simulink model "double_source_V3"  (R2023a)
settings: Solver=ode23tb  StartTime=0.0  StopTime=1  MaxStep=1e-6  RelTol=1e-3
libraries: spsSeriesRLCBranchLib x11, spsGroundLib x8, spsMosfetLib x8, spsVoltageMeasurementLib x4, spsACVoltageSourceLib x3, spsCurrentMeasurementLib x2, simulink x2, sps_lib x1
settings Model: Creator=25417  LastModifiedBy=25417

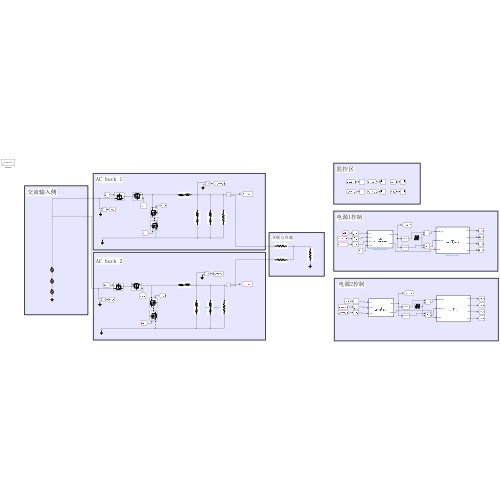
[thumbnail: Simulink's stored preview of the top-level diagram]
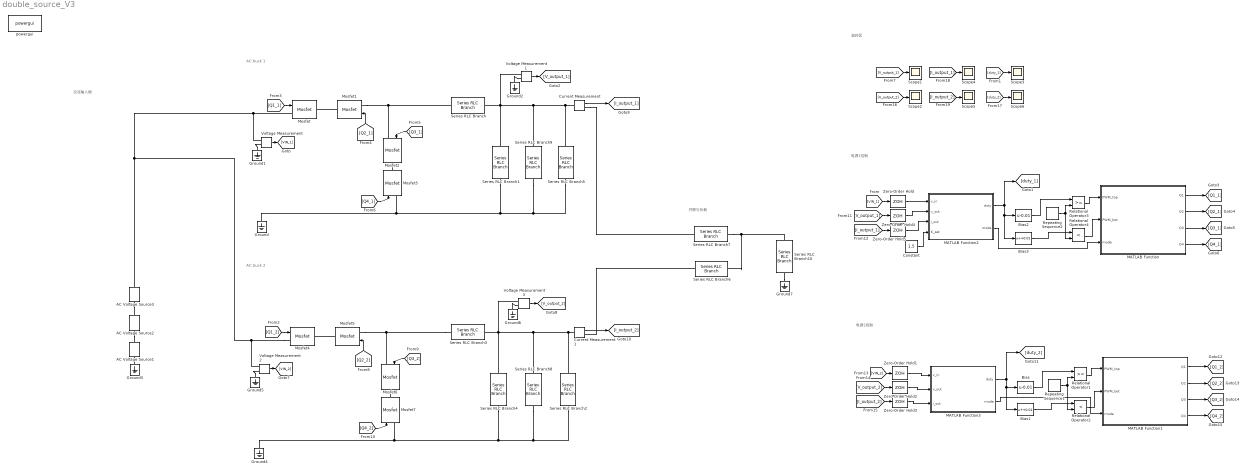
== system double_source_V3 ==
  note: 监控区
  note: 电源1控制
  note: 并联与负载
  note: AC buck 1
  note: 交流输入侧
  note: AC buck 2
  note: 电源2控制
  AC Voltage Source1 : spsACVoltageSourceLib/AC Voltage Source  Amplitude=70  Phase=0  Frequency=50  SampleTime=0  Measurements=None  BusType=swing  Pref=10e3  Qref=0  Qmin=-inf  Qmax=+inf
  AC Voltage Source2 : spsACVoltageSourceLib/AC Voltage Source  Amplitude=2.1  Phase=180  Frequency=150  SampleTime=0  Measurements=None  BusType=swing  Pref=10e3  Qref=0  Qmin=-inf  Qmax=+inf
  AC Voltage Source3 : spsACVoltageSourceLib/AC Voltage Source  Amplitude=1.4  Phase=180  Frequency=250  SampleTime=0  Measurements=None  BusType=swing  Pref=10e3  Qref=0  Qmin=-inf  Qmax=+inf
  Bias : Bias  Bias=-0.01  SaturateOnIntegerOverflow=off
  Bias1 : Bias  Bias=+0.01  SaturateOnIntegerOverflow=off
  Bias2 : Bias  Bias=-0.01  SaturateOnIntegerOverflow=off
  Bias3 : Bias  Bias=+0.01  SaturateOnIntegerOverflow=off
  Constant : Constant  Value=1.5
  Current Measurement : spsCurrentMeasurementLib/Current Measurement  PhasorSimulation=off  OutputType=Complex  PSBequivalent=0
  Current Measurement1 : spsCurrentMeasurementLib/Current Measurement  PhasorSimulation=off  OutputType=Complex  PSBequivalent=0
  Ground{,1..7} (8 alike) : spsGroundLib/Ground  LConnTagsString=a
  MATLAB Function : MATLAB Function  TreatAsAtomicUnit=on  SystemSampleTime=0
  MATLAB Function1 : MATLAB Function  TreatAsAtomicUnit=on  SystemSampleTime=0
  MATLAB Function2 : MATLAB Function  TreatAsAtomicUnit=on  SystemSampleTime=1/20e3
  MATLAB Function3 : MATLAB Function  TreatAsAtomicUnit=on  SystemSampleTime=1/20e3
  Mosfet{,1..7} (8 alike) : spsMosfetLib/Mosfet  Ron=0.1  Lon=0  Rd=0.01  Vfd=0  IC=0  Rs=1e5  Cs=inf  Measurements=off
  Relational Operator1 : RelationalOperator  OutDataTypeStr=boolean  RndMeth=Simplest  InputSameDT=off
  Relational Operator2 : RelationalOperator  Operator=<  OutDataTypeStr=boolean  RndMeth=Simplest  InputSameDT=off
  Relational Operator3 : RelationalOperator  OutDataTypeStr=boolean  RndMeth=Simplest  InputSameDT=off
  Relational Operator4 : RelationalOperator  Operator=<  OutDataTypeStr=boolean  RndMeth=Simplest  InputSameDT=off
  Repeating Sequence1 : simulink/Sources/Repeating Sequence  rep_seq_t=[0, 1/20000]  rep_seq_y=[0 1]
  Repeating Sequence2 : simulink/Sources/Repeating Sequence  rep_seq_t=[0, 1/20000]  rep_seq_y=[0 1]
  Scope{1..6} (6 alike) : Scope
  Series RLC Branch : spsSeriesRLCBranchLib/Series RLC Branch  LConnTagsString=__new0  RConnTagsString=__new0  BranchType=RL  Resistance=0.04  Inductance=450e-6  SetiL0=off  InitialCurrent=0  Capacitance=1e-6  Setx0=off  InitialVoltage=0  Measurements=None
  Series RLC Branch1 : spsSeriesRLCBranchLib/Series RLC Branch  LConnTagsString=__new0  RConnTagsString=__new0  BranchType=RC  Resistance=0.01  Inductance=1e-3  SetiL0=off  InitialCurrent=0  Capacitance=10.34e-6  Setx0=off  InitialVoltage=0  Measurements=None
  Series RLC Branch10 : spsSeriesRLCBranchLib/Series RLC Branch  LConnTagsString=__new0  RConnTagsString=__new0  BranchType=R  Resistance=10  Inductance=1e-3  SetiL0=off  InitialCurrent=0  Capacitance=10e-6  Setx0=off  InitialVoltage=0  Measurements=None
  Series RLC Branch2 : spsSeriesRLCBranchLib/Series RLC Branch  LConnTagsString=__new0  RConnTagsString=__new0  BranchType=R  Resistance=1.93e3  Inductance=1e-3  SetiL0=off  InitialCurrent=0  Capacitance=2e4  Setx0=off  InitialVoltage=0  Measurements=None
  Series RLC Branch3 : spsSeriesRLCBranchLib/Series RLC Branch  LConnTagsString=__new0  RConnTagsString=__new0  BranchType=RL  Resistance=0.07  Inductance=490e-6  SetiL0=off  InitialCurrent=0  Capacitance=1e-6  Setx0=off  InitialVoltage=0  Measurements=None
  Series RLC Branch4 : spsSeriesRLCBranchLib/Series RLC Branch  LConnTagsString=__new0  RConnTagsString=__new0  BranchType=RC  Resistance=0.01  Inductance=1e-3  SetiL0=off  InitialCurrent=0  Capacitance=9.54e-6  Setx0=off  InitialVoltage=0  Measurements=None
  Series RLC Branch5 : spsSeriesRLCBranchLib/Series RLC Branch  LConnTagsString=__new0  RConnTagsString=__new0  BranchType=R  Resistance=2.1e3  Inductance=1e-3  SetiL0=off  InitialCurrent=0  Capacitance=2e4  Setx0=off  InitialVoltage=0  Measurements=None
  Series RLC Branch6 : spsSeriesRLCBranchLib/Series RLC Branch  LConnTagsString=__new0  RConnTagsString=__new0  BranchType=R  Resistance=0.01  Inductance=1e-3  SetiL0=off  InitialCurrent=0  Capacitance=10e-6  Setx0=off  InitialVoltage=0  Measurements=None
  Series RLC Branch7 : spsSeriesRLCBranchLib/Series RLC Branch  LConnTagsString=__new0  RConnTagsString=__new0  BranchType=R  Resistance=0.01  Inductance=1e-3  SetiL0=off  InitialCurrent=0  Capacitance=10e-6  Setx0=off  InitialVoltage=0  Measurements=None
  Series RLC Branch8 : spsSeriesRLCBranchLib/Series RLC Branch  LConnTagsString=__new0  RConnTagsString=__new0  BranchType=RC  Resistance=0.01  Inductance=1e-3  SetiL0=off  InitialCurrent=0  Capacitance=4.5e-6  Setx0=off  InitialVoltage=0  Measurements=None
  Series RLC Branch9 : spsSeriesRLCBranchLib/Series RLC Branch  LConnTagsString=__new0  RConnTagsString=__new0  BranchType=RC  Resistance=0.01  Inductance=1e-3  SetiL0=off  InitialCurrent=0  Capacitance=4.81e-6  Setx0=off  InitialVoltage=0  Measurements=None
  Voltage Measurement{,1..3} (4 alike) : spsVoltageMeasurementLib/Voltage Measurement  PhasorSimulation=off  OutputType=Complex  PSBequivalent=0
  Zero-Order Hold{,1..5} (6 alike) : ZeroOrderHold  SampleTime=1/2e4
  powergui : sps_lib/powergui  Priority=1  SimulationMode=Continuous  SampleTime=5e-7  frequency=60  Iterations=50  frequencyindice=50  Pbase=100e6  ErrMax=1e-4  UnitsV=kV  UnitsW=MW  buscounter=0  FunctionMessages=off  echomessages=off  EnableUseOfTLC=off  CurrentSourceSwitches=off  DisableSnubberDevices=off  DisableRonSwitches=off  DisableVfSwitches=off  DisplayEquations=off  AutomaticDiscreteSolvers=off  SolverType=Tustin/Backward Euler (TBE)  Interpol=off  ExternalGateDelay=off  methode=off  Ts=100  x0status=blocks  SPID=on  SwTol=0  HookPort=off  NonlinearTolerance=1e-4  nMaxIteration=100  ContinueOnMaxIteration=off  RestoreLinks=warning  ResistiveCurrentMeasurement=off  Frange=[0:2:500]  Ylog=off  Xlog=on  ShowGrid=off  save=off  variable=ZData  structure=0  ZoomFFT=off  StartTime=0.0  cycles=1  DisplayStyle=1  fundamental=60  FreqAxis=off  MaxFrequency=1000  frequencyindicesteady=1  RmsSteady=1  display=off
  wires:
  Voltage Measurement/1 -> [VIN_1]
  [VIN_1] -> Zero-Order Hold/1
  Voltage Measurement1/1 -> [V_output_1]
  [Q1_1] -> Mosfet/1
  [Q2_1] -> Mosfet1/1
  [Q3_1] -> Mosfet2/1
  [Q4_1] -> Mosfet3/1
  [V_output_1] -> Scope1/1
  Zero-Order Hold/1 -> MATLAB Function2/1(v_in)
  [Q4_2] -> Mosfet7/1
  [Q3_2] -> Mosfet6/1
  [Q2_2] -> Mosfet5/1
  [Q1_2] -> Mosfet4/1
  Voltage Measurement3/1 -> [V_output_2]
  Voltage Measurement2/1 -> [VIN_2]
  Current Measurement/1 -> [I_output_1]
  Current Measurement1/1 -> [I_output_2]
  Relational Operator1/1 -> MATLAB Function1/1(PWM_top)
  Zero-Order Hold1/1 -> MATLAB Function3/1(v_in)
  [VIN_2] -> Zero-Order Hold1/1
  MATLAB Function3/1(duty) -> [duty_2], Bias1/1, Bias/1
  [V_output_2] -> Scope2/1
  [V_output_2] -> Zero-Order Hold2/1
  [I_output_2] -> Zero-Order Hold3/1
  Zero-Order Hold3/1 -> MATLAB Function3/3(i_out)
  Zero-Order Hold2/1 -> MATLAB Function3/2(v_out)
  [V_output_1] -> Zero-Order Hold4/1
  [I_output_1] -> Zero-Order Hold5/1
  Zero-Order Hold4/1 -> MATLAB Function2/2(v_out)
  Zero-Order Hold5/1 -> MATLAB Function2/3(i_out)
  [I_output_1] -> Scope4/1
  [I_output_2] -> Scope5/1
  [duty_1] -> Scope3/1
  [duty_2] -> Scope6/1
  Bias/1 -> Relational Operator1/1
  Bias1/1 -> Relational Operator2/1
  Repeating Sequence1/1 -> Relational Operator2/2, Relational Operator1/2
  Relational Operator2/1 -> MATLAB Function1/2(PWM_bot)
  MATLAB Function1/1(Q1) -> [Q1_2]
  MATLAB Function1/2(Q2) -> [Q2_2]
  MATLAB Function1/3(Q3) -> [Q3_2]
  MATLAB Function1/4(Q4) -> [Q4_2]
  Relational Operator4/1 -> MATLAB Function/2(PWM_bot)
  Bias2/1 -> Relational Operator3/1
  Bias3/1 -> Relational Operator4/1
  MATLAB Function2/1(duty) -> Bias3/1, Bias2/1, [duty_1]
  Repeating Sequence2/1 -> Relational Operator4/2, Relational Operator3/2
  Relational Operator3/1 -> MATLAB Function/1(PWM_top)
  MATLAB Function/1(Q1) -> [Q1_1]
  MATLAB Function/2(Q2) -> [Q2_1]
  MATLAB Function/3(Q3) -> [Q3_1]
  MATLAB Function/4(Q4) -> [Q4_1]
  MATLAB Function3/2(mode) -> MATLAB Function1/3(mode)
  MATLAB Function2/2(mode) -> MATLAB Function/3(mode)
  Constant/1 -> MATLAB Function2/4(K_set)
  connections:
  Mosfet1/RConn1 -- Mosfet/RConn1
  Mosfet1/LConn1 -- Mosfet2/LConn1 -- Series RLC Branch/LConn1
  Mosfet3/RConn1 -- Mosfet2/RConn1
  Mosfet3/LConn1 -- Series RLC Branch5/RConn1 -- Series RLC Branch9/RConn1 -- Series RLC Branch1/RConn1 -- Ground/LConn1
  Series RLC Branch1/LConn1 -- Current Measurement/LConn1 -- Series RLC Branch5/LConn1 -- Series RLC Branch9/LConn1 -- Voltage Measurement1/LConn1 -- Series RLC Branch/RConn1
  Voltage Measurement/LConn2 -- Ground1/LConn1
  Ground2/LConn1 -- Voltage Measurement1/LConn2
  Ground3/LConn1 -- AC Voltage Source1/LConn1
  Mosfet4/LConn1 -- Voltage Measurement2/LConn1 -- AC Voltage Source3/RConn1 -- Voltage Measurement/LConn1 -- Mosfet/LConn1
  Mosfet7/LConn1 -- Series RLC Branch2/RConn1 -- Series RLC Branch8/RConn1 -- Series RLC Branch4/RConn1 -- Ground4/LConn1
  Series RLC Branch3/LConn1 -- Mosfet5/LConn1 -- Mosfet6/LConn1
  Series RLC Branch4/LConn1 -- Series RLC Branch2/LConn1 -- Current Measurement1/LConn1 -- Series RLC Branch8/LConn1 -- Voltage Measurement3/LConn1 -- Series RLC Branch3/RConn1
  Voltage Measurement2/LConn2 -- Ground5/LConn1
  Mosfet7/RConn1 -- Mosfet6/RConn1
  Mosfet5/RConn1 -- Mosfet4/RConn1
  Ground6/LConn1 -- Voltage Measurement3/LConn2
  Series RLC Branch7/RConn1 -- Series RLC Branch10/LConn1 -- Series RLC Branch6/RConn1
  Series RLC Branch10/RConn1 -- Ground7/LConn1
  Current Measurement/RConn1 -- Series RLC Branch7/LConn1
  AC Voltage Source2/LConn1 -- AC Voltage Source1/RConn1
  AC Voltage Source3/LConn1 -- AC Voltage Source2/RConn1
  Series RLC Branch6/LConn1 -- Current Measurement1/RConn1

== matlab function double_source_V3/MATLAB Function1 ==
  data: Q1 output; PWM_top input; Q2 output; Q3 output; Q4 output; PWM_bot input; mode input
function [Q1, Q2, Q3, Q4] = Hardware_Router(PWM_top, PWM_bot, mode)
    pwm_t = double(PWM_top);
    pwm_b = double(PWM_bot);
    
    if mode == 1.0
        % ------------------------------------------------------
        % 正半周：打通下桥臂续流
        % ------------------------------------------------------
        Q1 = pwm_t;  
        Q2 = 1.0;    
        Q3 = pwm_b;  
        Q4 = 1.0;    
    elseif mode == -1.0
        % ------------------------------------------------------
        % 负半周：打通上桥臂续流
        % ------------------------------------------------------
        Q1 = 1.0;    
        Q2 = pwm_t;  
        Q3 = 1.0;    
        Q4 = pwm_b;  
    else
        % ------------------------------------------------------
        % 🌟 mode == 0.0：掉电封锁或死区跨越，全局安全关断
        % ------------------------------------------------------
        Q1 = 0.0;
        Q2 = 0.0;
        Q3 = 0.0;
        Q4 = 0.0;
    end
end

== matlab function double_source_V3/MATLAB Function ==
  data: Q1 output; PWM_top input; Q2 output; Q3 output; Q4 output; PWM_bot input; mode input
function [Q1, Q2, Q3, Q4] = Hardware_Router(PWM_top, PWM_bot, mode)
    pwm_t = double(PWM_top);
    pwm_b = double(PWM_bot);
    
    if mode == 1.0
        % ------------------------------------------------------
        % 正半周：打通下桥臂续流
        % ------------------------------------------------------
        Q1 = pwm_t;  
        Q2 = 1.0;    
        Q3 = pwm_b;  
        Q4 = 1.0;    
    elseif mode == -1.0
        % ------------------------------------------------------
        % 负半周：打通上桥臂续流
        % ------------------------------------------------------
        Q1 = 1.0;    
        Q2 = pwm_t;  
        Q3 = 1.0;    
        Q4 = pwm_b;  
    else
        % ------------------------------------------------------
        % 🌟 mode == 0.0：掉电封锁或死区跨越，全局安全关断
        % ------------------------------------------------------
        Q1 = 0.0;
        Q2 = 0.0;
        Q3 = 0.0;
        Q4 = 0.0;
    end
end

== matlab function double_source_V3/MATLAB Function2 ==
  data: v_in input; v_out input; i_out input; duty output; mode output; K_set input
function [duty, mode] = MCU_ISR_Master(v_in, v_out, i_out, K_set)
    % ==========================================================
    % [1] 用户接口与基础配置区
    % ==========================================================
    % 系统的绝对参考基准电压（有效值）
    % 设定值为后续所有调压、下垂计算的物理锚点。
    V_TARGET_RMS = 30.0; 
    
    % ==========================================================
    % [2] 闭环调参区
    % ==========================================================
    % 基础下垂系数：定义无通讯并联系统的基准输出阻抗
    % 主从机必须保持一致，它是电流反比分配定律的数学基石。
    BASE_DROOP    = 0.55;     
    
    % 电压 PI 环参数配置
    % 本架构属于“前馈主导 + PI辅助”的包络线控制。
    % 较低的比例(Kp)和积分(Ki)旨在只消除硬件线路(DCR/ESR)带来的稳态误差，
    % 避免由于强积分导致控制环路对谐波产生过激反应。
    KP_V          = 0.05;    
    KI_V          = 100.0;    
    
    % 硬件高频噪声低通滤波器系数 (用于平滑 ADC 原始采样值)
    ALPHA_LPF     = 0.35;    
    
    % SOGI 幅值校准系数，用于弥补离散化带来的轻微幅值衰减
    K_SOGI_SCALE  = 1.00;    
    
    % ==========================================================
    % [3] 内部静态变量声明区
    % ==========================================================
    % 声明 persistent 变量使其在每次中断进入时保持上一次的值
    
    % SOGI 提取输入电压的正交信号状态变量
    persistent v_alpha v_beta
    % SOGI 提取输出电压的正交信号状态变量
    persistent v_out_alpha v_out_beta 
    
    % PI 控制器的积分项与输出电压的低通滤波暂存值
    persistent pi_v_i v_out_f  
    % 状态机记忆变量与过零盲区计数器
    persistent last_mode zc_lock_cnt   
    
    % 主机专用的有功功率 IIR 低通滤波状态变量
    persistent p_avg 
    
    % 系统上电初始化逻辑
    if isempty(v_alpha)
        v_alpha = 0; v_beta = 0;
        p_avg = 0; pi_v_i = 0; v_out_f = 0; 
        v_out_alpha = 0; v_out_beta = 0; 
        last_mode = 0.0; 
        zc_lock_cnt = 0; 
    end
    
    % 采样周期与基波角频率定义 (基于 20kHz 中断频率与 50Hz 电网)
    Ts = 1/20000;             
    omega_0 = 2 * pi * 50;   
    k_sogi1 = 1.414; % SOGI 阻尼系数，决定带通滤波的带宽与响应速度
    
    % ==========================================================
    % [Step 1] 硬件级信号净化与输入电压 SOGI 提取
    % ==========================================================
    % 物理意义：ADC 采样的原始信号往往含有高频开关噪声，需要先进行简单的一阶低通滤波。
    % 随后，利用 SOGI (二阶广义积分器) 提取输入交流电的瞬时包络幅值。
    % 提取出的幅值用于前馈控制，能极大地削弱电网电压波动对输出的影响。
    
    v_out_f = (1 - ALPHA_LPF) * v_out_f + ALPHA_LPF * v_out;
    
    err_sogi = v_in - v_alpha;
    v_alpha = v_alpha + omega_0 * Ts * (k_sogi1 * err_sogi - v_beta);
    v_beta  = v_beta  + omega_0 * Ts * v_alpha; 
    v_in_amp = sqrt(v_alpha^2 + v_beta^2); 
    
    % ==========================================================
    % [Step 2] 状态机：交流欠压锁定与防抖过零检测
    % ==========================================================
    % 物理意义：逆变器需要根据输入电压的极性来切换桥臂的工作模式(正半周/负半周)。
    % 当输入源含有大量 3次、5次谐波时，过零点附近会出现多次极性反转（假过零）。
    % 这里的逻辑引入了 0.5V 的抗噪死区和 3ms 的软件盲区：
    % 一旦检测到真实的极性切换，强制锁定当前极性 3ms，无视期间的任何波动。
    
    GRID_OK = true;
    if v_in_amp < 15.0 
        GRID_OK = false;
    end
    
    if ~GRID_OK
        mode = 0.0; last_mode = 0.0; pi_v_i = 0.0; duty_raw = 0.0; zc_lock_cnt = 0;     
    else
        if zc_lock_cnt > 0
            % 处于过零盲区，维持上一周期的极性模式，倒数计数
            zc_lock_cnt = zc_lock_cnt - 1; mode = last_mode;
        else
            % 盲区外，执行带有 0.5V 迟滞的过零极性判定
            if last_mode <= 0.0 && v_in > 0.5
                mode = 1.0; zc_lock_cnt = 60; % 60次中断 * 50us = 3ms
            elseif last_mode >= 0.0 && v_in < -0.5
                mode = -1.0; zc_lock_cnt = 60; 
            else
                mode = last_mode;
            end
        end
        last_mode = mode;
    end
    
    % 防止后续作为分母时发生除以零的溢出错误
    if v_in_amp < 1.0; v_in_amp = 1.0; end 
    
    % ==========================================================
    % [Step 3] 输出电压 SOGI 提取有效值包络
    % ==========================================================
    % 物理意义：将 50Hz 的瞬时高频交流正弦波，转换为平缓的直流包络线标量。
    % 这一步将极其复杂的“交流波形跟踪控制”降维打击为简单的“直流稳压控制”，
    % 彻底消除了传统 PI 控制器跟踪正弦波时必然产生的相位滞后与幅值衰减。
    
    err_sogi_out = v_out_f - v_out_alpha;
    v_out_alpha = v_out_alpha + omega_0 * Ts * (k_sogi1 * err_sogi_out - v_out_beta);
    v_out_beta  = v_out_beta  + omega_0 * Ts * v_out_alpha;
    v_out_amp = sqrt(v_out_alpha^2 + v_out_beta^2) * K_SOGI_SCALE;
    
    % ==========================================================
    % [Step 4] 异构解耦核心：有功功率提取(IIR LPF)与动态下垂计算
    % ==========================================================
    % 物理意义与异构设计：
    % 畸变电网下，瞬时功率不仅含有直流量，还叠加了 100Hz、200Hz 等大量谐波脉动。
    % 主机采用了一阶 IIR 低通滤波器 (alpha_p = 0.010)。
    % 特性：它能像海绵一样平滑地吸收高频脉冲噪声，绝不产生阶跃突变。
    % 目的：让主机的下垂参考电压(v_ref_peak)呈现极度平滑的曲线，充当整个微电网中
    % 坚不可摧的“刚性电压源锚点”，从而在动态频域上与从机完全解耦。
    
    p_inst = v_out_f * i_out;
    alpha_p = 0.010; 
    p_avg = (1 - alpha_p) * p_avg + alpha_p * p_inst;
    i_active = p_avg / V_TARGET_RMS; 
    
    % 工程级防呆保护：防止设定的电流比例极小导致除法溢出
    if K_set < 0.1 
        K_set = 1.0; 
    end
    
    % 根据设定的分配比例 K_set 计算当前的动态下垂系数
    k_dynamic = BASE_DROOP / K_set;
    
    % 下垂控制核心公式：目标峰值电压 = 空载基准峰值 - 下垂阻抗压降
    V_nom_peak = V_TARGET_RMS * 1.414; 
    v_ref_peak = V_nom_peak - k_dynamic * i_active;
    
    if v_ref_peak < 0; v_ref_peak = 0; end
    if v_ref_peak > 50.0; v_ref_peak = 50.0; end 
    
    % ==========================================================
    % [Step 5] 闭环控制：前馈占空比合成与 PI 误差修正
    % ==========================================================
    % 物理意义：
    % 1. 物理前馈 (duty_ff)：直接利用输出目标值除以输入母线值。这一步完成了
    %    95% 的控制任务，使得系统即便没有 PI 也能给出大致准确的波形。
    % 2. 误差补偿 (duty_pi)：PI 控制器仅负责消除由于硬件电感 DCR、走线电阻
    %    以及前馈计算误差带来的几百毫伏的残余压差。
    
    if mode == 0.0
        duty_raw = 0.0;
    else
        % 计算包络线的直流误差
        err_amp = v_ref_peak - v_out_amp; 
        
        pi_v_p = KP_V * err_amp;
        pi_v_i = pi_v_i + KI_V * err_amp * Ts;
        
        % 积分器抗饱和限幅 (Anti-Windup)
        % 防止在空载切满载的瞬间，积分器过度累积导致后续巨大的电压超调
        if pi_v_i > 25.0; pi_v_i = 25.0; elseif pi_v_i < -25.0; pi_v_i = -25.0; end
        
        % 标幺化合成：补偿项 + 物理前馈项
        duty_pi = (pi_v_p + pi_v_i) / v_in_amp; 
        duty_ff = v_ref_peak / v_in_amp; 
        
        duty_raw = duty_ff + duty_pi;
        
        % 硬件级物理限幅：防止 PWM 发出全开或全关信号导致桥臂直通失控
        if duty_raw > 0.99
            duty_raw = 0.99; 
        elseif duty_raw < 0.01  
            duty_raw = 0.0; 
        end
    end
    
    duty = double(duty_raw);
end

== matlab function double_source_V3/MATLAB Function3 ==
  data: v_in input; v_out input; i_out input; duty output; mode output
function [duty, mode] = MCU_ISR_Slave(v_in, v_out, i_out)
    % ==========================================================
    % [1] 用户接口与基础配置区
    % ==========================================================
    % 从机的物理电压锚点，必须与主机严格对称
    V_TARGET_RMS = 30.0; 
    
    % ==========================================================
    % [2] 闭环调参区
    % ==========================================================
    % 固定下垂系数
    % 从机不接受外部比例调节，仅依靠此参数自主响应有功功率变化
    BASE_DROOP    = 0.55;     
    KP_V          = 0.05;    
    KI_V          = 100.0;    
    ALPHA_LPF     = 0.35;    
    K_SOGI_SCALE  = 1.00;    
    
    % ==========================================================
    % [3] 内部静态变量声明区
    % ==========================================================
    persistent v_alpha v_beta
    persistent pi_v_i v_out_f  
    persistent v_out_alpha v_out_beta 
    persistent last_mode
    persistent zc_lock_cnt   
    
    % 从机专用的功率滑动平均滤波 (MAF) 环形缓冲数组与索引
    persistent p_buf p_idx 
    
    if isempty(v_alpha)
        v_alpha = 0; v_beta = 0;
        pi_v_i = 0; v_out_f = 0; 
        v_out_alpha = 0; v_out_beta = 0; 
        last_mode = 0.0; 
        zc_lock_cnt = 0; 
        
        % 数组长度 200。在 20kHz 采样率下，200次中断 = 10ms 时间窗口
        % 10ms 正好对应 50Hz 交流瞬时功率中 100Hz(偶次) 纹波的一个完整周期
        p_buf = zeros(200, 1); 
        p_idx = 1;
    end
    
    Ts = 1/20000;             
    omega_0 = 2 * pi * 50;   
    k_sogi1 = 1.414; 
    
    % ==========================================================
    % [Step 1] 硬件级信号净化与输入电压 SOGI 提取
    % ==========================================================
    v_out_f = (1 - ALPHA_LPF) * v_out_f + ALPHA_LPF * v_out;
    
    err_sogi = v_in - v_alpha;
    v_alpha = v_alpha + omega_0 * Ts * (k_sogi1 * err_sogi - v_beta);
    v_beta  = v_beta  + omega_0 * Ts * v_alpha; 
    v_in_amp = sqrt(v_alpha^2 + v_beta^2); 
    
    % ==========================================================
    % [Step 2] 状态机：交流欠压锁定与防抖过零检测
    % ==========================================================
    GRID_OK = true;
    if v_in_amp < 15.0 
        GRID_OK = false;
    end
    
    if ~GRID_OK
        mode = 0.0; last_mode = 0.0; pi_v_i = 0.0; duty_raw = 0.0; zc_lock_cnt = 0;     
    else
        if zc_lock_cnt > 0
            zc_lock_cnt = zc_lock_cnt - 1; mode = last_mode;
        else
            if last_mode <= 0.0 && v_in > 0.5
                mode = 1.0; zc_lock_cnt = 60; 
            elseif last_mode >= 0.0 && v_in < -0.5
                mode = -1.0; zc_lock_cnt = 60; 
            else
                mode = last_mode;
            end
        end
        last_mode = mode;
    end
    
    if v_in_amp < 1.0; v_in_amp = 1.0; end 
    
    % ==========================================================
    % [Step 3] 输出电压 SOGI 提取有效值包络
    % ==========================================================
    err_sogi_out = v_out_f - v_out_alpha;
    v_out_alpha = v_out_alpha + omega_0 * Ts * (k_sogi1 * err_sogi_out - v_out_beta);
    v_out_beta  = v_out_beta  + omega_0 * Ts * v_out_alpha;
    v_out_amp = sqrt(v_out_alpha^2 + v_out_beta^2) * K_SOGI_SCALE;
    
    % ==========================================================
    % [Step 4] 异构解耦核心：有功功率提取(FIR MAF)与固定下垂控制
    % ==========================================================
    % 物理意义与异构设计：
    % 从机采用了基于长度为 10ms 滑动窗口的 MAF 滤波器。
    % 特性：它在频域上天然具备针对 100Hz 的陷波极点，能彻底剔除纹波，
    % 但会在时域上产生固定延迟的微观突变。
    % 目的：从机甘当“迟钝的跟随者”。它无视瞬态的谐波干扰，只针对绝对的纯直流
    % 有功功率进行下垂均流响应。即便 MAF 的微观突变会在参考电压上产生锯齿，
    % 但因为已被主机(LPF)的刚性源化解，两者不会发生共振，实现了极佳的系统鲁棒性。
    
    p_inst = v_out_f * i_out;
    
    % 维护滑动数据窗口
    p_buf(p_idx) = p_inst;
    p_idx = p_idx + 1;
    if p_idx > 200
        p_idx = 1;
    end
    
    % 求取 10ms 内的平均有功功率，并转化为等效有功电流
    p_avg = sum(p_buf) / 200.0; 
    i_active = p_avg / V_TARGET_RMS; 
    
    % 执行固定下垂阻抗策略
    V_nom_peak = V_TARGET_RMS * 1.414; 
    v_ref_peak = V_nom_peak - BASE_DROOP * i_active;
    
    if v_ref_peak < 0; v_ref_peak = 0; end
    if v_ref_peak > 50.0; v_ref_peak = 50.0; end 
    
    % ==========================================================
    % [Step 5] 闭环控制：前馈占空比合成与 PI 误差修正
    % ==========================================================
    if mode == 0.0
        duty_raw = 0.0;
    else
        err_amp = v_ref_peak - v_out_amp; 
        
        pi_v_p = KP_V * err_amp;
        pi_v_i = pi_v_i + KI_V * err_amp * Ts;
        
        if pi_v_i > 25.0; pi_v_i = 25.0; elseif pi_v_i < -25.0; pi_v_i = -25.0; end
        
        duty_pi = (pi_v_p + pi_v_i) / v_in_amp; 
        duty_ff = v_ref_peak / v_in_amp; 
        
        duty_raw = duty_ff + duty_pi;
        
        if duty_raw > 0.99
            duty_raw = 0.99; 
        elseif duty_raw < 0.01  
            duty_raw = 0.0; 
        end
    end
    
    duty = double(duty_raw);
end
